simulink model "osservatore_1"  (R2019b)
settings: Solver=VariableStepAuto  StartTime=0.0  StopTime=10.0  MaxStep=1e-3  RelTol=1e-3
undefined symbols (not defined in the file): A, B, C, L
libraries: cstblocks x1
settings Model: Creator=jacobi  LastModifiedBy=manue

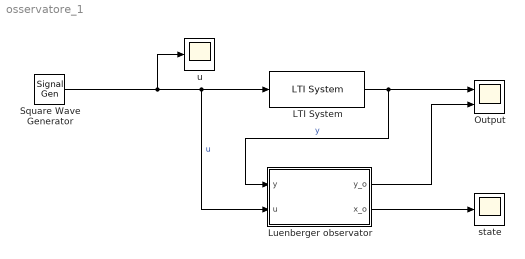
== system osservatore_1 ==
  LTI System : cstblocks/LTI System  sys=P  IC=[]
  Luenberger observator : Subsystem
  Output : Scope  NumInputPorts=2
  Square Wave Generator : SignalGenerator  WaveForm=square  Units=rad/sec
  state : Scope
  u : Scope
  wires:
  LTI System/1 -> Output/1, Luenberger observator/1(y)  "y"
  Square Wave Generator/1 -> u/1, Luenberger observator/2(u), LTI System/1  "u"
  Luenberger observator/1(y_o) -> Output/2
  Luenberger observator/2(x_o) -> state/1

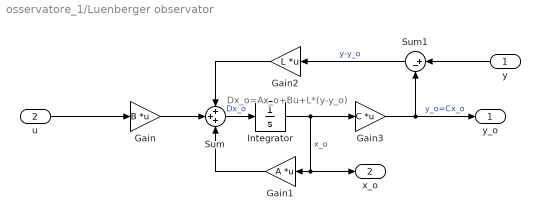
== system osservatore_1/Luenberger observator ==
  note: Dx_o=Ax_o+Bu+L*(y-y_o)
  y : Inport
  u : Inport  Port=2
  Gain : Gain  Gain=B  Multiplication=Matrix(K*u)
  Gain1 : Gain  Gain=A  Multiplication=Matrix(K*u)
  Gain2 : Gain  Gain=L  Multiplication=Matrix(K*u)
  Gain3 : Gain  Gain=C  Multiplication=Matrix(K*u)
  Integrator : Integrator
  Sum : Sum  Inputs=+++
  Sum1 : Sum  Inputs=|+-
  y_o : Outport
  x_o : Outport  Port=2
  wires:
  Integrator/1 -> Gain3/1, x_o/1, Gain1/1  "x_o"
  Sum/1 -> Integrator/1  "Dx_o"
  Gain1/1 -> Sum/3
  Gain/1 -> Sum/2
  Gain3/1 -> Sum1/2, y_o/1  "y_o=Cx_o"
  Sum1/1 -> Gain2/1  "y-y_o"
  Gain2/1 -> Sum/1
  u/1 -> Gain/1
  y/1 -> Sum1/1
